simulink library "atlas_impctrl_library"  (Simulink 8.5)
settings: Solver=ode45  StartTime=0.0  StopTime=10.0  RelTol=1e-3
values from neighbouring files (symbols this model uses):
  B = d - 0.1*ones(NJL,1)    [atlas_joint_impctrl_sqrt_damping_test_settings_default.m]
  D = 0.7*eye(NJL)    [atlas_joint_impctrl_sqrt_damping_test_settings_default.m]
  K_d = 150*eye(NJL)    [atlas_joint_impctrl_sqrt_damping_test_settings_default.m]
  K_ext_c = 0    [atlas_joint_impctrl_sqrt_damping_test_settings_default.m]
  K_ext_o = 1    [atlas_joint_impctrl_sqrt_damping_test_settings_default.m]
  K_fri_o = 1    [atlas_joint_impctrl_sqrt_damping_test_settings_default.m]
  K_O = 5*eye(NJL)    [atlas_joint_impctrl_sqrt_damping_test_settings_default.m]
  K_obs_c = 0    [atlas_joint_impctrl_sqrt_damping_test_settings_default.m]
  K_qD_d = 1    [atlas_joint_impctrl_sqrt_damping_test_settings_default.m]
  K_qDD_d = 1    [atlas_joint_impctrl_sqrt_damping_test_settings_default.m]
  K_tau_a = 1    [atlas_joint_impctrl_sqrt_damping_test_settings_default.m]
  K_tau_c = 1    [atlas_joint_impctrl_sqrt_damping_test_settings_default.m]
  K_tau_D = 1    [atlas_joint_impctrl_sqrt_damping_test_settings_default.m]
  K_tau_e = 0    [atlas_joint_impctrl_sqrt_damping_test_settings_default.m]
  K_tau_f = 0    [atlas_joint_impctrl_sqrt_damping_test_settings_default.m]
  K_tau_g = 1    [atlas_joint_impctrl_sqrt_damping_test_settings_default.m]
  K_tau_K = 1    [atlas_joint_impctrl_sqrt_damping_test_settings_default.m]
  K_tau_o = 0    [atlas_joint_impctrl_sqrt_damping_test_settings_default.m]
  qD_th = 0.05*ones(NJL,1)    [atlas_joint_impctrl_sqrt_damping_test_settings_default.m]
  T = 0.001    [atlas_joint_impctrl_sqrt_damping_test_settings_default.m]
  T1 = 0    [atlas_joint_impctrl_sqrt_damping_test_settings_default.m]
  tau_c = muC - 4*ones(NJL,1)    [atlas_joint_impctrl_sqrt_damping_test_settings_default.m]
  tau_th = 0.02*ones(NJL,1)    [atlas_joint_impctrl_sqrt_damping_test_settings_default.m]
undefined symbols (not defined in the file or in its folder): K_tau_F, mr, offsets
undefined symbols (not defined in the file): atlas_arm_lr, atlas_leg_lr, delta_s, MPV, MPV_arm_damp, MPV_arm_model, MPV_leg_damp, MPV_leg_model, qD_s, tau_s
libraries: atlas_dynamic_library x23, atlas_impctrl_library x18, dspmtrx3 x3
(part 1 of 2)
settings Model: Creator=knoechelmann  LastModifiedBy=schappler  CovSFcnEnable=off

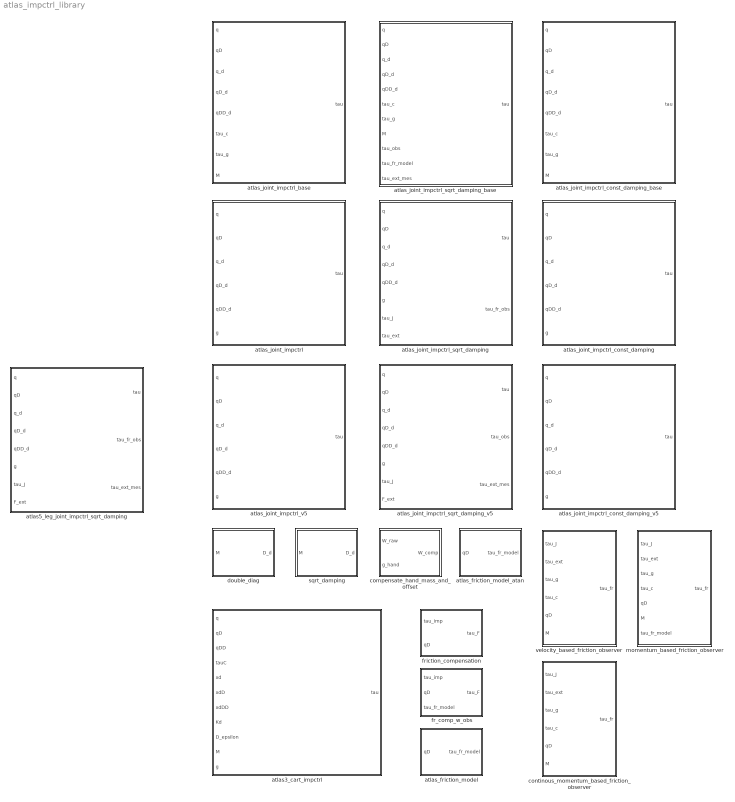
== system atlas_impctrl_library ==
  atlas3_cart_impctrl : Subsystem  TreatAsAtomicUnit=on
  atlas5_leg_joint_impctrl_sqrt_damping : Subsystem  TreatAsAtomicUnit=on  SystemSampleTime=T  mask(Atlas Joint Impedance Controller){K_d=K_d, D=D, K_tau_g=K_tau_g, K_tau_c=K_tau_c, K_tau_K=K_tau_K, K_tau_D=K_tau_D, K_tau_a=K_tau_a, K_tau_f=K_tau_f, K_tau_e=K_tau_e, K_tau_o=K_tau_o, K_qD_d=K_qD_d, K_qDD_d=K_qDD_d, K_ext_c=K_ext_c, K_obs_c=K_obs_c, K_fri_o=K_fri_o, K_ext_o=K_ext_o, tau_obs_max=30*ones(6,1), MPV_leg_damp=MPV_leg_damp, MPV_leg_model=MPV_leg_model, tau_c=tau_c, B=B, qD_th=qD_th, tau_th=tau_th, K_O=K_O, T=T, atlas_leg_lr=atlas_leg_lr, T1=T1}
      mask prompts: K_d "K_d (desired stiffness)"; D "D (diagonal matrix with desired damping coefficients)"; K_tau_g "K_tau_g (gain of gravity compensation)"; K_tau_c "K_tau_c (gain of corriolis- and inertia compensation)"; K_tau_K "K_tau_K (gain of stiffness component)"; K_tau_D "K_tau_D (gain of damping component)"; K_tau_a "K_tau_a (gain of acceleration component)"; K_tau_f "K_tau_f (gain of friction compensation)"; K_tau_e "K_tau_e (gain of external torque)"; K_tau_o "K_tau_o (gain of compensation of disturbance observer torques)"; K_qD_d "K_qD_d (gain of desired velocity)"; K_qDD_d "K_qDD_d (gain of desired acceleration)"; K_ext_c "K_ext_c (input gain to deside, wether to trigger friction compensation via the measured external torque)"; K_obs_c "K_obs_c (input gain to deside, wether to trigger friction compensation via the observed torque)"; K_fri_o "K_fri_o (input gain of friction model torques for observer)"; K_ext_o "K_ext_o (input gain of external torque for observer)"; tau_obs_max "tau_obs_max (limit for observed disturbance torque)"; MPV_leg_damp "MPV_damp (base parameter vector for damping calculation)"; MPV_leg_model "MPV_model (base parameter vector for dynamic model calculation)"; tau_c "tau_c (vector with coulomb friction momentums for all joints)"; B "B (vector with viscous friction coefficients of all joints)"; qD_th "qD_th (vector with theshold velocities for stiction)"; tau_th "tau_th (vector with kick-in momentums for stiction compensation)"; K_O "K_O (friction observer gain)"; T "T (sample time (important for friction observer))"; atlas_leg_lr "atlas_leg_lr (left/right flag)"; T1 "T1 (low pass filter time constant for inertia matrix)"
      mask help:
      | Hardware dependent full impedance controller block with matrix
      | squareroot damping design for the atlas robot. For a better
      | testing, all partial momentums can be individually scaled.
      | Coulomb-, viscous friction and Stribeck stiction is taken into
      | account for friction compensation.
  atlas_friction_model : Subsystem  TreatAsAtomicUnit=on  mask{tau_c=tau_c, B=B}
      mask prompts: tau_c "tau_c (vector with coulomb friction momentums for all joints)"; B "B (vector with viscous friction coefficients of all joints)"
  atlas_friction_model_atan : Subsystem  TreatAsAtomicUnit=on  mask{tau_c=tau_c, B=B}
      mask prompts: tau_c "tau_c (vector with coulomb friction momentums for all joints)"; B "B (vector with viscous friction coefficients of all joints)"
  atlas_joint_impctrl : Subsystem  TreatAsAtomicUnit=on  mask(Atlas Joint Impedance Controller){K_d=K_d, D=D, tau_c=tau_c, B=B, tau_s=tau_s, qD_s=qD_s, delta_s=delta_s, qD_th=qD_th, tau_th=tau_th, K_tau_g=K_tau_g, K_tau_c=K_tau_c, K_tau_F=K_tau_F, K_tau_K=K_tau_K, K_tau_D=K_tau_D, K_tau_a=K_tau_a, MPV=MPV}
      mask prompts: K_d "K_d (desired stiffness)"; D "D (diagonal matrix with desired damping coefficients)"; tau_c "tau_c (vector with coulomb friction momentums for all joints)"; B "B (vector with viscous friction coefficients of all joints)"; tau_s "tau_s (vector with sticition momentums of all joints)"; qD_s "qD_s (vector with Stribeck velocities of all joints)"; delta_s "delta_s (vector with stiction exponents for all joints)"; qD_th "qD_th (vector with theshold velocities for stiction)"; tau_th "tau_th (vector with kick-in momentums for stiction compensation)"; K_tau_g "K_tau_g (gain of gravity compensation)"; K_tau_c "K_tau_c (gain of corriolis- and inertia compensation)"; K_tau_F "K_tau_F (gain of friction compensation)"; K_tau_K "K_tau_K (gain of stiffness component)"; K_tau_D "K_tau_D (gain of damping component)"; K_tau_a "K_tau_a (gain of acceleration component)"; MPV "MPV (vector of minimal parameters)"
      mask help:
      | Hardware dependent full impedance controller block with matrix
      | double diagonalization damping design for the atlas robot. For
      | a better testing, all partial momentums can be individually
      | scaled. Coulomb-, viscous friction and Stribeck stiction is taken
      | into account for friction compensation.
  atlas_joint_impctrl_base : Subsystem  TreatAsAtomicUnit=on  mask(Joint Impedance Controller Base){K_d=K_d, D=D, tau_c=tau_c, B=B, tau_s=tau_s, qD_s=qD_s, delta_s=delta_s, qD_th=qD_th, tau_th=tau_th, K_tau_g=K_tau_g, K_tau_c=K_tau_c, K_tau_F=K_tau_F, K_tau_K=K_tau_K, K_tau_D=K_tau_D, K_tau_a=K_tau_a}
      mask prompts: K_d "K_d (desired stiffness)"; D "D (diagonal matrix with desired damping coefficients)"; tau_c "tau_c (vector with coulomb friction momentums for all joints)"; B "B (vector with viscous friction coefficients of all joints)"; tau_s "tau_s (vector with sticition momentums of all joints)"; qD_s "qD_s (vector with Stribeck velocities of all joints)"; delta_s "delta_s (vector with stiction exponents for all joints)"; qD_th "qD_th (vector with theshold velocities for stiction)"; tau_th "tau_th (vector with kick-in momentums for stiction compensation)"; K_tau_g "K_tau_g (gain of gravity compensation)"; K_tau_c "K_tau_c (gain of corriolis- and inertia compensation)"; K_tau_F "K_tau_F (gain of friction compensation)"; K_tau_K "K_tau_K (gain of stiffness component)"; K_tau_D "K_tau_D (gain of damping component)"; K_tau_a "K_tau_a (gain of acceleration component)"
      mask help:
      | Hardware independent impedance controller base block with mdouble
      | diagonalization damping design. For a better testing, all partial
      | momentums can be individually scaled. Coulomb-, viscous friction
      | and Stribeck stiction is taken into account for friction compen-
      | sation.
  atlas_joint_impctrl_const_damping : Subsystem  TreatAsAtomicUnit=on  mask(Atlas Joint Impedance Controller){K_d=K_d, D=D, tau_c=tau_c, B=B, tau_s=tau_s, qD_s=qD_s, delta_s=delta_s, qD_th=qD_th, tau_th=tau_th, K_tau_g=K_tau_g, K_tau_c=K_tau_c, K_tau_F=K_tau_F, K_tau_K=K_tau_K, K_tau_D=K_tau_D, K_tau_a=K_tau_a, MPV=MPV}
      mask prompts: K_d "K_d (desired stiffness)"; D "D (diagonal matrix with desired damping coefficients)"; tau_c "tau_c (vector with coulomb friction momentums for all joints)"; B "B (vector with viscous friction coefficients of all joints)"; tau_s "tau_s (vector with sticition momentums of all joints)"; qD_s "qD_s (vector with Stribeck velocities of all joints)"; delta_s "delta_s (vector with stiction exponents for all joints)"; qD_th "qD_th (vector with theshold velocities for stiction)"; tau_th "tau_th (vector with kick-in momentums for stiction compensation)"; K_tau_g "K_tau_g (gain of gravity compensation)"; K_tau_c "K_tau_c (gain of corriolis- and inertia compensation)"; K_tau_F "K_tau_F (gain of friction compensation)"; K_tau_K "K_tau_K (gain of stiffness component)"; K_tau_D "K_tau_D (gain of damping component)"; K_tau_a "K_tau_a (gain of acceleration component)"; MPV "MPV (vector of minimal parameters)"
      mask help:
      | Hardware dependent full impedance controller block with
      | constant damping design for the atlas robot. For a better
      | testing, all partial momentums can be individually scaled.
      | Coulomb-, viscous friction and Stribeck stiction is taken into
      | account for friction compensation.
  atlas_joint_impctrl_const_damping_base : Subsystem  TreatAsAtomicUnit=on  mask(Joint Impedance Controller Base){K_d=K_d, D=D, tau_c=tau_c, B=B, tau_s=tau_s, qD_s=qD_s, delta_s=delta_s, qD_th=qD_th, tau_th=tau_th, K_tau_g=K_tau_g, K_tau_c=K_tau_c, K_tau_F=K_tau_F, K_tau_K=K_tau_K, K_tau_D=K_tau_D, K_tau_a=K_tau_a}
      mask prompts: K_d "K_d (desired stiffness)"; D "D (diagonal matrix with desired damping coefficients)"; tau_c "tau_c (vector with coulomb friction momentums for all joints)"; B "B (vector with viscous friction coefficients of all joints)"; tau_s "tau_s (vector with sticition momentums of all joints)"; qD_s "qD_s (vector with Stribeck velocities of all joints)"; delta_s "delta_s (vector with stiction exponents for all joints)"; qD_th "qD_th (vector with theshold velocities for stiction)"; tau_th "tau_th (vector with kick-in momentums for stiction compensation)"; K_tau_g "K_tau_g (gain of gravity compensation)"; K_tau_c "K_tau_c (gain of corriolis- and inertia compensation)"; K_tau_F "K_tau_F (gain of friction compensation)"; K_tau_K "K_tau_K (gain of stiffness component)"; K_tau_D "K_tau_D (gain of damping component)"; K_tau_a "K_tau_a (gain of acceleration component)"
      mask help:
      | Hardware independent impedance controller base block with constant
      | damping design. For a better testing, all partial momentums can be
      | individually scaled. Coulomb-, viscous friction and Stribeck stiction
      | is taken into account for friction compensation.
  atlas_joint_impctrl_const_damping_v5 : Subsystem  TreatAsAtomicUnit=on  mask(Atlas Joint Impedance Controller){K_d=K_d, D=D, tau_c=tau_c, B=B, tau_s=tau_s, qD_s=qD_s, delta_s=delta_s, qD_th=qD_th, tau_th=tau_th, K_tau_g=K_tau_g, K_tau_c=K_tau_c, K_tau_F=K_tau_F, K_tau_K=K_tau_K, K_tau_D=K_tau_D, K_tau_a=K_tau_a, MPV=MPV}
      mask prompts: K_d "K_d (desired stiffness)"; D "D (diagonal matrix with desired damping coefficients)"; tau_c "tau_c (vector with coulomb friction momentums for all joints)"; B "B (vector with viscous friction coefficients of all joints)"; tau_s "tau_s (vector with sticition momentums of all joints)"; qD_s "qD_s (vector with Stribeck velocities of all joints)"; delta_s "delta_s (vector with stiction exponents for all joints)"; qD_th "qD_th (vector with theshold velocities for stiction)"; tau_th "tau_th (vector with kick-in momentums for stiction compensation)"; K_tau_g "K_tau_g (gain of gravity compensation)"; K_tau_c "K_tau_c (gain of corriolis- and inertia compensation)"; K_tau_F "K_tau_F (gain of friction compensation)"; K_tau_K "K_tau_K (gain of stiffness component)"; K_tau_D "K_tau_D (gain of damping component)"; K_tau_a "K_tau_a (gain of acceleration component)"; MPV "MPV (vector of minimal parameters)"
      mask help:
      | Hardware dependent full impedance controller block with
      | constant damping design for the atlas robot. For a better
      | testing, all partial momentums can be individually scaled.
      | Coulomb-, viscous friction and Stribeck stiction is taken into
      | account for friction compensation.
  atlas_joint_impctrl_sqrt_damping : Subsystem  TreatAsAtomicUnit=on  mask(Atlas Joint Impedance Controller){K_d=K_d, D=D, K_tau_g=K_tau_g, K_tau_c=K_tau_c, K_tau_K=K_tau_K, K_tau_D=K_tau_D, K_tau_a=K_tau_a, K_qD_d=K_qD_d, K_qDD_d=K_qDD_d, MPV=MPV, K_O=K_O, T=T}
      mask prompts: K_d "K_d (desired stiffness)"; D "D (diagonal matrix with desired damping coefficients)"; K_tau_g "K_tau_g (gain of gravity compensation)"; K_tau_c "K_tau_c (gain of corriolis- and inertia compensation)"; K_tau_K "K_tau_K (gain of stiffness component)"; K_tau_D "K_tau_D (gain of damping component)"; K_tau_a "K_tau_a (gain of acceleration component)"; K_qD_d "K_qD_d (gain of desired velocity)"; K_qDD_d "K_qDD_d (gain of desired acceleration)"; MPV "MPV (vector of minimal parameters)"; K_O "K_O (friction observer gain)"; T "T (sample time (important for friction observer))"
      mask help:
      | Hardware dependent full impedance controller block with matrix
      | squareroot damping design for the atlas robot. For a better
      | testing, all partial momentums can be individually scaled.
      | Coulomb-, viscous friction and Stribeck stiction is taken into
      | account for friction compensation.
  atlas_joint_impctrl_sqrt_damping_base : Subsystem  TreatAsAtomicUnit=on  mask(Joint Impedance Controller Base){K_d=K_d, D=D, K_tau_g=K_tau_g, K_tau_c=K_tau_c, K_tau_K=K_tau_K, K_tau_D=K_tau_D, K_tau_a=K_tau_a, K_tau_f=K_tau_f, K_tau_e=K_tau_e, K_tau_o=K_tau_o, K_qD_d=K_qD_d, K_qDD_d=K_qDD_d, K_ext_c=K_ext_c, K_obs_c=K_obs_c, tau_c=tau_c, B=B, qD_th=qD_th, tau_th=tau_th}
      mask prompts: K_d "K_d (desired stiffness)"; D "D (diagonal matrix with desired damping coefficients)"; K_tau_g "K_tau_g (gain of gravity compensation)"; K_tau_c "K_tau_c (gain of corriolis- and inertia compensation)"; K_tau_K "K_tau_K (gain of stiffness component)"; K_tau_D "K_tau_D (gain of damping component)"; K_tau_a "K_tau_a (gain of acceleration component)"; K_tau_f "K_tau_f (gain of model based friction compensation)"; K_tau_e "K_tau_e (gain of compensation of external torque measurd via hand sensor)"; K_tau_o "K_tau_o (gain of compensation of disturbance observer torques)"; K_qD_d "K_qD_d (gain of desired velocity)"; K_qDD_d "K_qDD_d (gain of desired acceleration)"; K_ext_c "K_ext_c (input gain to deside, wether to trigger friction compensation via the measured external torque)"; K_obs_c "K_obs_c (input gain to deside, wether to trigger friction compensation via the observed torque)"; tau_c "tau_c (vector with coulomb friction momentums for all joints)"; B "B (vector with viscous friction coefficients of all joints)"; qD_th "qD_th (vector with theshold velocities for stiction)"; tau_th "tau_th (vector with kick-in momentums for stiction compensation)"
      mask help:
      | Hardware independent impedance controller base block with matrix
      | squareroot damping design. For a better testing, all partial mo-
      | mentums can be individually scaled. Coulomb-, viscous friction
      | and Stribeck stiction is taken into account for friction compen-
      | sation.
  atlas_joint_impctrl_sqrt_damping_v5 : Subsystem  TreatAsAtomicUnit=on  SystemSampleTime=T  mask(Atlas Joint Impedance Controller){K_d=K_d, D=D, K_tau_g=K_tau_g, K_tau_c=K_tau_c, K_tau_K=K_tau_K, K_tau_D=K_tau_D, K_tau_a=K_tau_a, K_tau_f=K_tau_f, K_tau_e=K_tau_e, K_tau_o=K_tau_o, K_qD_d=K_qD_d, K_qDD_d=K_qDD_d, K_ext_c=K_ext_c, K_obs_c=K_obs_c, K_fri_o=K_fri_o, K_ext_o=K_ext_o, tau_obs_max=30*ones(7,1), MPV_arm_damp=MPV_arm_damp, MPV_arm_model=MPV_arm_model, tau_c=tau_c, B=B, qD_th=qD_th, tau_th=tau_th, K_O=K_O, T=T, atlas_arm_lr=atlas_arm_lr, T1=T1}
      mask prompts: K_d "K_d (desired stiffness)"; D "D (diagonal matrix with desired damping coefficients)"; K_tau_g "K_tau_g (gain of gravity compensation)"; K_tau_c "K_tau_c (gain of corriolis- and inertia compensation)"; K_tau_K "K_tau_K (gain of stiffness component)"; K_tau_D "K_tau_D (gain of damping component)"; K_tau_a "K_tau_a (gain of acceleration component)"; K_tau_f "K_tau_f (gain of model based friction compensation)"; K_tau_e "K_tau_e (gain of compensation of external torque measurd via hand sensor)"; K_tau_o "K_tau_o (gain of compensation of disturbance observer torques)"; K_qD_d "K_qD_d (gain of desired velocity)"; K_qDD_d "K_qDD_d (gain of desired acceleration)"; K_ext_c "K_ext_c (input gain to deside, wether to trigger friction compensation via the measured external torque)"; K_obs_c "K_obs_c (input gain to deside, wether to trigger friction compensation via the observed torque)"; K_fri_o "K_fri_o (input gain of friction model torques for observer)"; K_ext_o "K_ext_o (input gain of external torque for observer)"; tau_obs_max "tau_obs_max (limit for observed disturbance torque)"; MPV_arm_damp "MPV_damp (base parameter vector for damping calculation)"; MPV_arm_model "MPV_model (base parameter vector for dynamic model calculation)"; tau_c "tau_c (vector with coulomb friction momentums for all joints)"; B "B (vector with viscous friction coefficients of all joints)"; qD_th "qD_th (vector with theshold velocities for stiction)"; tau_th "tau_th (vector with kick-in momentums for stiction compensation)"; K_O "K_O (friction observer gain)"; T "T (sample time (important for friction observer))"; atlas_arm_lr "atlas_arm_lr (flag for left or right side)"; T1 "T1 (low pass filter time constant for inertia matrix)"
      mask help:
      | Hardware dependent full impedance controller block with matrix
      | squareroot damping design for the atlas robot. For a better
      | testing, all partial momentums can be individually scaled.
      | Coulomb-, viscous friction and Stribeck stiction is taken into
      | account for friction compensation.
  atlas_joint_impctrl_v5 : Subsystem  TreatAsAtomicUnit=on  mask(Atlas Joint Impedance Controller){K_d=K_d, D=D, tau_c=tau_c, B=B, tau_s=tau_s, qD_s=qD_s, delta_s=delta_s, qD_th=qD_th, tau_th=tau_th, K_tau_g=K_tau_g, K_tau_c=K_tau_c, K_tau_F=K_tau_F, K_tau_K=K_tau_K, K_tau_D=K_tau_D, K_tau_a=K_tau_a, MPV=MPV}
      mask prompts: K_d "K_d (desired stiffness)"; D "D (diagonal matrix with desired damping coefficients)"; tau_c "tau_c (vector with coulomb friction momentums for all joints)"; B "B (vector with viscous friction coefficients of all joints)"; tau_s "tau_s (vector with sticition momentums of all joints)"; qD_s "qD_s (vector with Stribeck velocities of all joints)"; delta_s "delta_s (vector with stiction exponents for all joints)"; qD_th "qD_th (vector with theshold velocities for stiction)"; tau_th "tau_th (vector with kick-in momentums for stiction compensation)"; K_tau_g "K_tau_g (gain of gravity compensation)"; K_tau_c "K_tau_c (gain of corriolis- and inertia compensation)"; K_tau_F "K_tau_F (gain of friction compensation)"; K_tau_K "K_tau_K (gain of stiffness component)"; K_tau_D "K_tau_D (gain of damping component)"; K_tau_a "K_tau_a (gain of acceleration component)"; MPV "MPV (vector of minimal parameters)"
      mask help:
      | Hardware dependent full impedance controller block with matrix
      | double diagonalization damping design for the atlas robot. For
      | a better testing, all partial momentums can be individually
      | scaled. Coulomb-, viscous friction and Stribeck stiction is taken
      | into account for friction compensation.
  compensate_hand_mass_and_offset : Subsystem  TreatAsAtomicUnit=on  mask{mr=mr, Parameter2offsets=offsets}
      mask prompts: mr "mr (mass (1) and com  (2-4) of the hand in hand frame)"; Parameter2offsets "offsets (sensor offsets of F/T-sensor)"
  continous_momentum_based_friction_observer : Subsystem  TreatAsAtomicUnit=on  mask{K_O=K_O}
      mask prompts: K_O "K_O (Observer gain)"
  double_diag : Subsystem  TreatAsAtomicUnit=on  mask{K_d=K_d, D=D}
  fr_comp_w_obs : Subsystem  TreatAsAtomicUnit=on  mask{tau_c=tau_c, B=B, qD_th=qD_th, tau_th=tau_th}
      mask prompts: tau_c "tau_c (vector with coulomb friction momentums for all joints)"; B "B (vector with viscous friction coefficients of all joints)"; qD_th "qD_th (vector with theshold velocities for stiction)"; tau_th "tau_th (vector with kick-in momentums for stiction compensation)"
  friction_compensation : Subsystem  TreatAsAtomicUnit=on  mask{tau_c=tau_c, B=B, qD_th=qD_th, tau_th=tau_th}
      mask prompts: tau_c "tau_c (vector with coulomb friction momentums for all joints)"; B "B (vector with viscous friction coefficients of all joints)"; qD_th "qD_th (vector with theshold velocities for stiction)"; tau_th "tau_th (vector with kick-in momentums for stiction compensation)"
  momentum_based_friction_observer : Subsystem  TreatAsAtomicUnit=on  SystemSampleTime=T  mask{K_O=K_O, T=T, T1=T1, tau_out_max=30*ones(6,1)}
      mask prompts: K_O "K_O (Observer gain)"; T "T (sampletime)"; T1 "T1 (low pass differentiator time constant)"; tau_out_max "tau_out_max (safety limit for output, output will be limited to lie in between -tau_out_max and tau_out_max)"
  sqrt_damping : Subsystem  TreatAsAtomicUnit=on  mask{K_d=K_d, D=D}
  velocity_based_friction_observer : Subsystem  TreatAsAtomicUnit=on  mask{K_O=K_O, T=T}
      mask prompts: K_O "K_O (Observer gain)"; T "T (sampletime)"

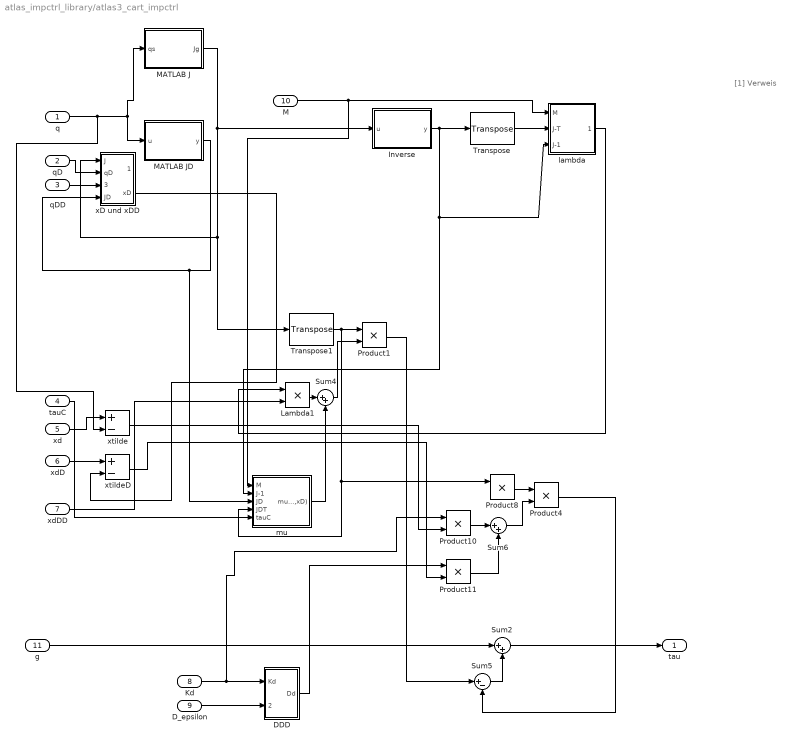
== system atlas_impctrl_library/atlas3_cart_impctrl ==
  note: [1] Verweis
  q : Inport
  qD : Inport  Port=2
  qDD : Inport  Port=3
  tauC : Inport  Port=4
  xd : Inport  Port=5
  xdD : Inport  Port=6
  xdDD : Inport  Port=7
  Kd : Inport  Port=8
  D_epsilon : Inport  Port=9
  M : Inport  Port=10
  g : Inport  Port=11
  DDD : Subsystem
  Inverse : MATLAB Function  TreatAsAtomicUnit=on
  Lambda1 : Product
  MATLAB J : MATLAB Function  TreatAsAtomicUnit=on
  MATLAB JD : MATLAB Function  TreatAsAtomicUnit=on
  Product{1,4,8,10..11} (5 alike) : Product
  Sum2 : Sum  Inputs=|++
  Sum4 : Sum  Inputs=|++
  Sum5 : Sum  Inputs=|+-
  Sum6 : Sum  Inputs=|++
  Transpose : dspmtrx3/Transpose  Hermitian=off  overflowFlag=off
  Transpose1 : dspmtrx3/Transpose  Hermitian=off  overflowFlag=off
  lambda : Subsystem
  mu : Subsystem
  xD und xDD : Subsystem
  xtilde : Sum  Inputs=+-
  xtildeD : Sum  Inputs=+-
  tau : Outport
  wires:
  DDD/1(Dd) -> Product11/1
  Product10/1 -> Sum6/1
  Product8/1 -> Product4/1
  xdD/1 -> xtildeD/1
  Transpose1/1 -> Product8/1, mu/4(JDT), Product1/1
  Product4/1 -> Sum5/2
  Product11/1 -> Sum6/2
  Sum2/1 -> tau/1
  Inverse/1(y) -> mu/2(J-1), lambda/3(J-1), Transpose/1
  g/1 -> Sum2/1
  Sum6/1 -> Product4/2
  M/1 -> mu/1(M), lambda/1(M)
  MATLAB J/1(Jg) -> xD und xDD/1(J), Transpose1/1, Inverse/1(u)
  xd/1 -> xtilde/1
  xtilde/1 -> Product10/2
  MATLAB JD/1(y) -> mu/3(JD), xD und xDD/4(JD)
  Sum4/1 -> Product1/2
  Sum5/1 -> Sum2/2
  Lambda1/1 -> Sum4/1
  xdDD/1 -> Lambda1/2
  q/1 -> MATLAB J/1(qs), MATLAB JD/1(u), xtilde/2
  xtildeD/1 -> Product11/2
  Product1/1 -> Sum5/1
  lambda/1(Lambda) -> Lambda1/1
  Transpose/1 -> lambda/2(J-T)
  tauC/1 -> mu/5(tauC)
  mu/1(mu(x,xD)) -> Sum4/2
  qD/1 -> xD und xDD/2(qD)
  qDD/1 -> xD und xDD/3(qDD)
  xD und xDD/2(xD) -> xtildeD/2
  Kd/1 -> Product10/1, DDD/1(Kd)
  D_epsilon/1 -> DDD/2(D_epsilon)

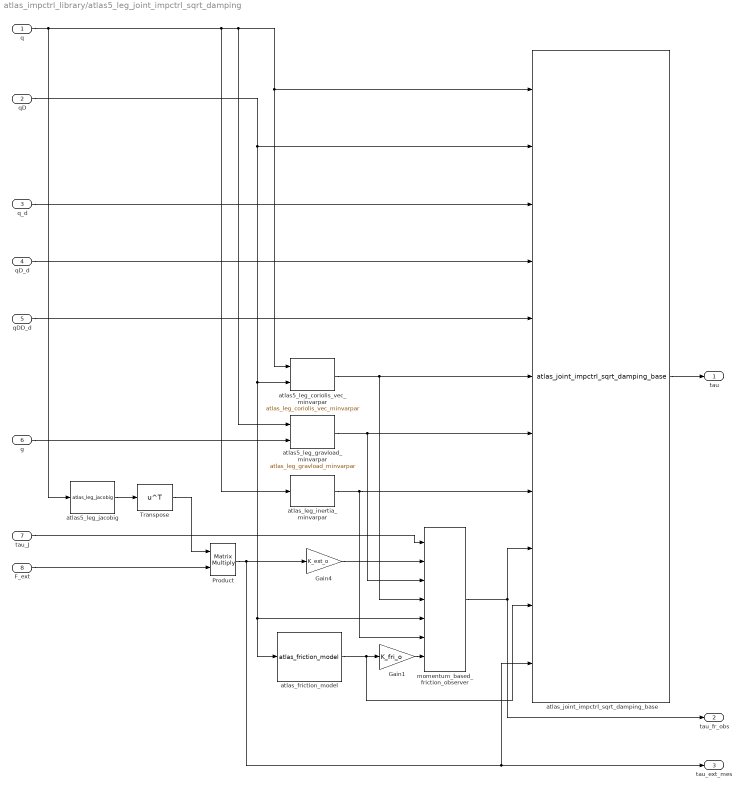
== system atlas_impctrl_library/atlas5_leg_joint_impctrl_sqrt_damping ==
  q : Inport  OutDataTypeStr=double  PortDimensions=6
  qD : Inport  Port=2  OutDataTypeStr=double  PortDimensions=6
  q_d : Inport  Port=3  OutDataTypeStr=double  PortDimensions=6
  qD_d : Inport  Port=4  OutDataTypeStr=double  PortDimensions=6
  qDD_d : Inport  Port=5  OutDataTypeStr=double  PortDimensions=6
  g : Inport  Port=6  OutDataTypeStr=double  PortDimensions=[3 1]
  tau_J : Inport  Port=7  OutDataTypeStr=double  PortDimensions=6
  F_ext : Inport  Port=8  OutDataTypeStr=double  PortDimensions=6
  Gain1 : Gain  Gain=K_fri_o
  Gain4 : Gain  Gain=K_ext_o
  Product : Product  Multiplication=Matrix(*)
  Transpose : Math  Operator=transpose  SaturateOnIntegerOverflow=on
  atlas5_leg_coriolis_vec_minvarpar : atlas_dynamic_library/atlas_leg_coriolis_vec_minvarpar  atlas_arm_lr=atlas_leg_lr  atlas_version=uint8(5)  MPV=MPV_leg_model
  atlas5_leg_gravload_minvarpar : atlas_dynamic_library/atlas_leg_gravload_minvarpar  atlas_arm_lr=atlas_leg_lr  atlas_version=uint8(5)  MPV=MPV_leg_model
  atlas5_leg_jacobig : atlas_dynamic_library/atlas_leg_jacobig  atlas_version=uint8(5)  atlas_leg_lr=atlas_leg_lr
  atlas_friction_model : atlas_impctrl_library/atlas_friction_model  tau_c=tau_c  B=B
  atlas_joint_impctrl_sqrt_damping_base : atlas_impctrl_library/atlas_joint_impctrl_sqrt_damping_base  K_d=K_d  D=D  K_tau_g=K_tau_g  K_tau_c=K_tau_c  K_tau_K=K_tau_K  K_tau_D=K_tau_D  K_tau_a=K_tau_a  K_tau_f=K_tau_f  K_tau_e=K_tau_e  K_tau_o=K_tau_o  K_qD_d=K_qD_d  K_qDD_d=K_qDD_d  K_ext_c=K_ext_c  K_obs_c=K_obs_c  tau_c=tau_c  B=B  qD_th=qD_th  tau_th=tau_th
  atlas_leg_inertia_minvarpar : atlas_dynamic_library/atlas_leg_inertia_minvarpar  atlas_arm_lr=atlas_leg_lr  atlas_version=uint8(5)  MPV=MPV_leg_damp
  momentum_based_friction_observer : atlas_impctrl_library/momentum_based_friction_observer  K_O=K_O  T=T  T1=T1  tau_out_max=tau_obs_max
  tau : Outport  OutDataTypeStr=double  PortDimensions=6
  tau_fr_obs : Outport  Port=2  OutDataTypeStr=double  PortDimensions=6
  tau_ext_mes : Outport  Port=3  OutDataTypeStr=double  PortDimensions=6
  wires:
  atlas_joint_impctrl_sqrt_damping_base/1 -> tau/1
  atlas_leg_inertia_minvarpar/1 -> atlas_joint_impctrl_sqrt_damping_base/8, momentum_based_friction_observer/6
  q/1 -> atlas_joint_impctrl_sqrt_damping_base/1, atlas5_leg_coriolis_vec_minvarpar/1, atlas5_leg_gravload_minvarpar/1, atlas_leg_inertia_minvarpar/1, atlas5_leg_jacobig/1
  qD/1 -> atlas_joint_impctrl_sqrt_damping_base/2, atlas5_leg_coriolis_vec_minvarpar/2, momentum_based_friction_observer/5, atlas_friction_model/1
  q_d/1 -> atlas_joint_impctrl_sqrt_damping_base/3
  atlas5_leg_coriolis_vec_minvarpar/1 -> atlas_joint_impctrl_sqrt_damping_base/6, momentum_based_friction_observer/4
  qD_d/1 -> atlas_joint_impctrl_sqrt_damping_base/4
  atlas5_leg_gravload_minvarpar/1 -> atlas_joint_impctrl_sqrt_damping_base/7, momentum_based_friction_observer/3
  qDD_d/1 -> atlas_joint_impctrl_sqrt_damping_base/5
  g/1 -> atlas5_leg_gravload_minvarpar/2
  momentum_based_friction_observer/1 -> tau_fr_obs/1, atlas_joint_impctrl_sqrt_damping_base/9
  tau_J/1 -> momentum_based_friction_observer/1
  atlas5_leg_jacobig/1 -> Transpose/1
  Transpose/1 -> Product/1
  F_ext/1 -> Product/2
  Product/1 -> atlas_joint_impctrl_sqrt_damping_base/11, tau_ext_mes/1, Gain4/1
  Gain4/1 -> momentum_based_friction_observer/2
  atlas_friction_model/1 -> atlas_joint_impctrl_sqrt_damping_base/10, Gain1/1
  Gain1/1 -> momentum_based_friction_observer/7

== system atlas_impctrl_library/atlas_friction_model ==
  qD : Inport
  atlas_friction_model : MATLAB Function  TreatAsAtomicUnit=on
  tau_fr_model : Outport
  wires:
  qD/1 -> atlas_friction_model/1(qD)
  atlas_friction_model/1(tau_fr_model) -> tau_fr_model/1

== system atlas_impctrl_library/atlas_friction_model_atan ==
  qD : Inport
  atlas_friction_model_atan : MATLAB Function  TreatAsAtomicUnit=on
  tau_fr_model : Outport
  wires:
  qD/1 -> atlas_friction_model_atan/1(qD)
  atlas_friction_model_atan/1(tau_fr_model) -> tau_fr_model/1

== system atlas_impctrl_library/atlas_joint_impctrl ==
  q : Inport
  qD : Inport  Port=2
  q_d : Inport  Port=3
  qD_d : Inport  Port=4
  qDD_d : Inport  Port=5
  g : Inport  Port=6
  atlas_arm_coriolis_vec_minvarpar : atlas_dynamic_library/atlas_arm_coriolis_vec_minvarpar  atlas_arm_lr=atlas_arm_lr  atlas_version=atlas_version  MPV=MPV
  atlas_arm_gravload_minvarpar : atlas_dynamic_library/atlas_arm_gravload_minvarpar  atlas_arm_lr=atlas_arm_lr  atlas_version=atlas_version  MPV=MPV
  atlas_arm_inertia_minvarpar : atlas_dynamic_library/atlas_arm_inertia_minvarpar  atlas_arm_lr=atlas_arm_lr  atlas_version=atlas_version  MPV=MPV
  atlas_joint_impctrl_base : atlas_impctrl_library/atlas_joint_impctrl_base  K_d=K_d  D=D  tau_c=tau_c  B=B  tau_s=tau_s  qD_s=qD_s  delta_s=delta_s  qD_th=qD_th  tau_th=tau_th  K_tau_g=K_tau_g  K_tau_c=K_tau_c  K_tau_F=K_tau_F  K_tau_K=K_tau_K  K_tau_D=K_tau_D  K_tau_a=K_tau_a
  tau : Outport
  wires:
  atlas_joint_impctrl_base/1 -> tau/1
  atlas_arm_inertia_minvarpar/1 -> atlas_joint_impctrl_base/8
  q/1 -> atlas_arm_inertia_minvarpar/1, atlas_arm_gravload_minvarpar/1, atlas_joint_impctrl_base/1, atlas_arm_coriolis_vec_minvarpar/1
  qD/1 -> atlas_joint_impctrl_base/2, atlas_arm_coriolis_vec_minvarpar/2
  q_d/1 -> atlas_joint_impctrl_base/3
  atlas_arm_coriolis_vec_minvarpar/1 -> atlas_joint_impctrl_base/6
  qD_d/1 -> atlas_joint_impctrl_base/4
  atlas_arm_gravload_minvarpar/1 -> atlas_joint_impctrl_base/7
  qDD_d/1 -> atlas_joint_impctrl_base/5
  g/1 -> atlas_arm_gravload_minvarpar/2

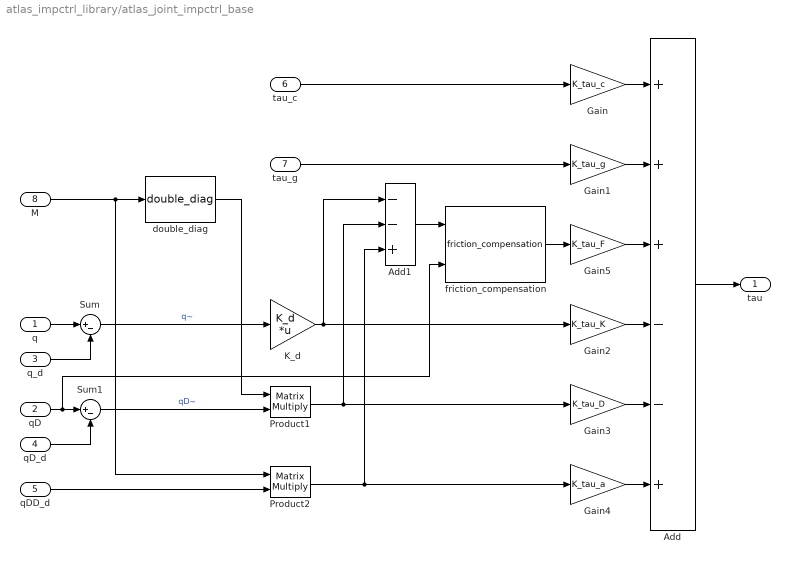
== system atlas_impctrl_library/atlas_joint_impctrl_base ==
  q : Inport
  qD : Inport  Port=2
  q_d : Inport  Port=3
  qD_d : Inport  Port=4
  qDD_d : Inport  Port=5
  tau_c : Inport  Port=6
  tau_g : Inport  Port=7
  M : Inport  Port=8
  Add : Sum  Inputs=+++--+
  Add1 : Sum  Inputs=--+
  Gain : Gain  Gain=K_tau_c
  Gain1 : Gain  Gain=K_tau_g
  Gain2 : Gain  Gain=K_tau_K
  Gain3 : Gain  Gain=K_tau_D
  Gain4 : Gain  Gain=K_tau_a
  Gain5 : Gain  Gain=K_tau_F
  K_d : Gain  Gain=K_d  Multiplication=Matrix(K*u)
  Product1 : Product  Multiplication=Matrix(*)
  Product2 : Product  Multiplication=Matrix(*)
  Sum : Sum  Inputs=|+-
  Sum1 : Sum  Inputs=|+-
  double_diag : atlas_impctrl_library/double_diag  K_d=K_d  D=D
  friction_compensation : atlas_impctrl_library/friction_compensation  tau_c=tau_c  B=B  qD_th=qD_th  tau_th=tau_th
  tau : Outport
  wires:
  M/1 -> double_diag/1, Product2/1
  q/1 -> Sum/1
  q_d/1 -> Sum/2
  qD/1 -> friction_compensation/2, Sum1/1
  qD_d/1 -> Sum1/2
  Sum1/1 -> Product1/2  "qD~"
  Sum/1 -> K_d/1  "q~"
  qDD_d/1 -> Product2/2
  double_diag/1 -> Product1/1
  Add/1 -> tau/1
  K_d/1 -> Add1/1, Gain2/1
  tau_g/1 -> Gain1/1
  tau_c/1 -> Gain/1
  Product1/1 -> Add1/2, Gain3/1
  Product2/1 -> Add1/3, Gain4/1
  Gain/1 -> Add/1
  Gain1/1 -> Add/2
  Gain2/1 -> Add/4
  Gain3/1 -> Add/5
  Gain4/1 -> Add/6
  Gain5/1 -> Add/3
  friction_compensation/1 -> Gain5/1
  Add1/1 -> friction_compensation/1

== system atlas_impctrl_library/atlas_joint_impctrl_const_damping ==
  q : Inport
  qD : Inport  Port=2
  q_d : Inport  Port=3
  qD_d : Inport  Port=4
  qDD_d : Inport  Port=5
  g : Inport  Port=6
  atlas_arm_coriolis_vec_minvarpar : atlas_dynamic_library/atlas_arm_coriolis_vec_minvarpar  atlas_arm_lr=atlas_arm_lr  atlas_version=atlas_version  MPV=MPV
  atlas_arm_gravload_minvarpar : atlas_dynamic_library/atlas_arm_gravload_minvarpar  atlas_arm_lr=atlas_arm_lr  atlas_version=atlas_version  MPV=MPV
  atlas_arm_inertia_minvarpar : atlas_dynamic_library/atlas_arm_inertia_minvarpar  atlas_arm_lr=atlas_arm_lr  atlas_version=atlas_version  MPV=MPV
  atlas_joint_impctrl_const_damping_base : atlas_impctrl_library/atlas_joint_impctrl_const_damping_base  K_d=K_d  D=D  tau_c=tau_c  B=B  tau_s=tau_s  qD_s=qD_s  delta_s=delta_s  qD_th=qD_th  tau_th=tau_th  K_tau_g=K_tau_g  K_tau_c=K_tau_c  K_tau_F=K_tau_F  K_tau_K=K_tau_K  K_tau_D=K_tau_D  K_tau_a=K_tau_a
  tau : Outport
  wires:
  atlas_joint_impctrl_const_damping_base/1 -> tau/1
  atlas_arm_inertia_minvarpar/1 -> atlas_joint_impctrl_const_damping_base/8
  q/1 -> atlas_arm_inertia_minvarpar/1, atlas_arm_gravload_minvarpar/1, atlas_joint_impctrl_const_damping_base/1, atlas_arm_coriolis_vec_minvarpar/1
  qD/1 -> atlas_joint_impctrl_const_damping_base/2, atlas_arm_coriolis_vec_minvarpar/2
  q_d/1 -> atlas_joint_impctrl_const_damping_base/3
  atlas_arm_coriolis_vec_minvarpar/1 -> atlas_joint_impctrl_const_damping_base/6
  qD_d/1 -> atlas_joint_impctrl_const_damping_base/4
  atlas_arm_gravload_minvarpar/1 -> atlas_joint_impctrl_const_damping_base/7
  qDD_d/1 -> atlas_joint_impctrl_const_damping_base/5
  g/1 -> atlas_arm_gravload_minvarpar/2

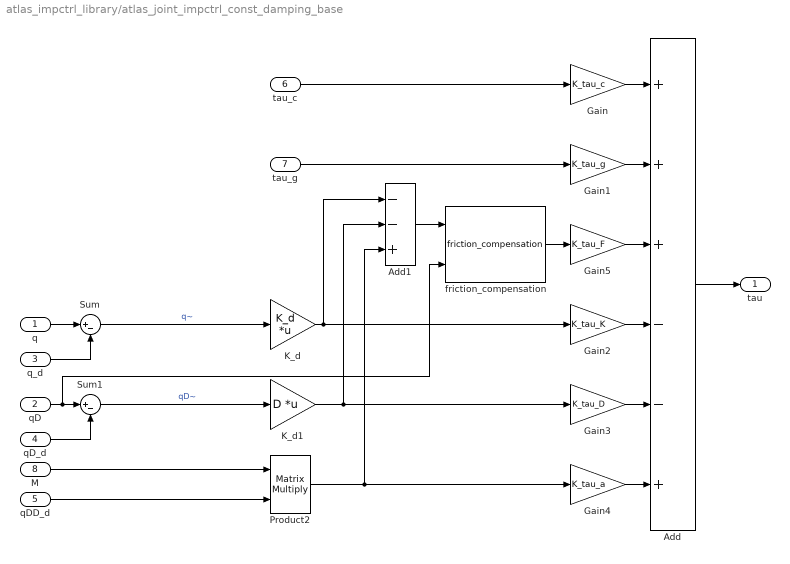
== system atlas_impctrl_library/atlas_joint_impctrl_const_damping_base ==
  q : Inport
  qD : Inport  Port=2
  q_d : Inport  Port=3
  qD_d : Inport  Port=4
  qDD_d : Inport  Port=5
  tau_c : Inport  Port=6
  tau_g : Inport  Port=7
  M : Inport  Port=8
  Add : Sum  Inputs=+++--+
  Add1 : Sum  Inputs=--+
  Gain : Gain  Gain=K_tau_c
  Gain1 : Gain  Gain=K_tau_g
  Gain2 : Gain  Gain=K_tau_K
  Gain3 : Gain  Gain=K_tau_D
  Gain4 : Gain  Gain=K_tau_a
  Gain5 : Gain  Gain=K_tau_F
  K_d : Gain  Gain=K_d  Multiplication=Matrix(K*u)
  K_d1 : Gain  Gain=D  Multiplication=Matrix(K*u)
  Product2 : Product  Multiplication=Matrix(*)
  Sum : Sum  Inputs=|+-
  Sum1 : Sum  Inputs=|+-
  friction_compensation : atlas_impctrl_library/friction_compensation  tau_c=tau_c  B=B  qD_th=qD_th  tau_th=tau_th
  tau : Outport
  wires:
  M/1 -> Product2/1
  q/1 -> Sum/1
  q_d/1 -> Sum/2
  qD/1 -> friction_compensation/2, Sum1/1
  qD_d/1 -> Sum1/2
  Sum1/1 -> K_d1/1  "qD~"
  Sum/1 -> K_d/1  "q~"
  qDD_d/1 -> Product2/2
  Add/1 -> tau/1
  K_d/1 -> Add1/1, Gain2/1
  tau_g/1 -> Gain1/1
  tau_c/1 -> Gain/1
  K_d1/1 -> Add1/2, Gain3/1
  Product2/1 -> Add1/3, Gain4/1
  Gain/1 -> Add/1
  Gain1/1 -> Add/2
  Gain2/1 -> Add/4
  Gain3/1 -> Add/5
  Gain4/1 -> Add/6
  Gain5/1 -> Add/3
  friction_compensation/1 -> Gain5/1
  Add1/1 -> friction_compensation/1

== system atlas_impctrl_library/atlas_joint_impctrl_const_damping_v5 ==
  q : Inport
  qD : Inport  Port=2
  q_d : Inport  Port=3
  qD_d : Inport  Port=4
  qDD_d : Inport  Port=5
  g : Inport  Port=6
  atlas_arm_coriolis_vec_minvarpar : atlas_dynamic_library/atlas_arm_coriolis_vec_minvarpar  atlas_arm_lr=atlas_arm_lr  atlas_version=atlas_version  MPV=MPV
  atlas_arm_gravload_minvarpar : atlas_dynamic_library/atlas_arm_gravload_minvarpar  atlas_arm_lr=atlas_arm_lr  atlas_version=atlas_version  MPV=MPV
  atlas_arm_inertia_minvarpar : atlas_dynamic_library/atlas_arm_inertia_minvarpar  atlas_arm_lr=atlas_arm_lr  atlas_version=atlas_version  MPV=MPV
  atlas_joint_impctrl_const_damping_base : atlas_impctrl_library/atlas_joint_impctrl_const_damping_base  K_d=K_d  D=D  tau_c=tau_c  B=B  tau_s=tau_s  qD_s=qD_s  delta_s=delta_s  qD_th=qD_th  tau_th=tau_th  K_tau_g=K_tau_g  K_tau_c=K_tau_c  K_tau_F=K_tau_F  K_tau_K=K_tau_K  K_tau_D=K_tau_D  K_tau_a=K_tau_a
  tau : Outport
  wires:
  atlas_joint_impctrl_const_damping_base/1 -> tau/1
  atlas_arm_inertia_minvarpar/1 -> atlas_joint_impctrl_const_damping_base/8
  q/1 -> atlas_arm_inertia_minvarpar/1, atlas_arm_gravload_minvarpar/1, atlas_joint_impctrl_const_damping_base/1, atlas_arm_coriolis_vec_minvarpar/1
  qD/1 -> atlas_joint_impctrl_const_damping_base/2, atlas_arm_coriolis_vec_minvarpar/2
  q_d/1 -> atlas_joint_impctrl_const_damping_base/3
  atlas_arm_coriolis_vec_minvarpar/1 -> atlas_joint_impctrl_const_damping_base/6
  qD_d/1 -> atlas_joint_impctrl_const_damping_base/4
  atlas_arm_gravload_minvarpar/1 -> atlas_joint_impctrl_const_damping_base/7
  qDD_d/1 -> atlas_joint_impctrl_const_damping_base/5
  g/1 -> atlas_arm_gravload_minvarpar/2

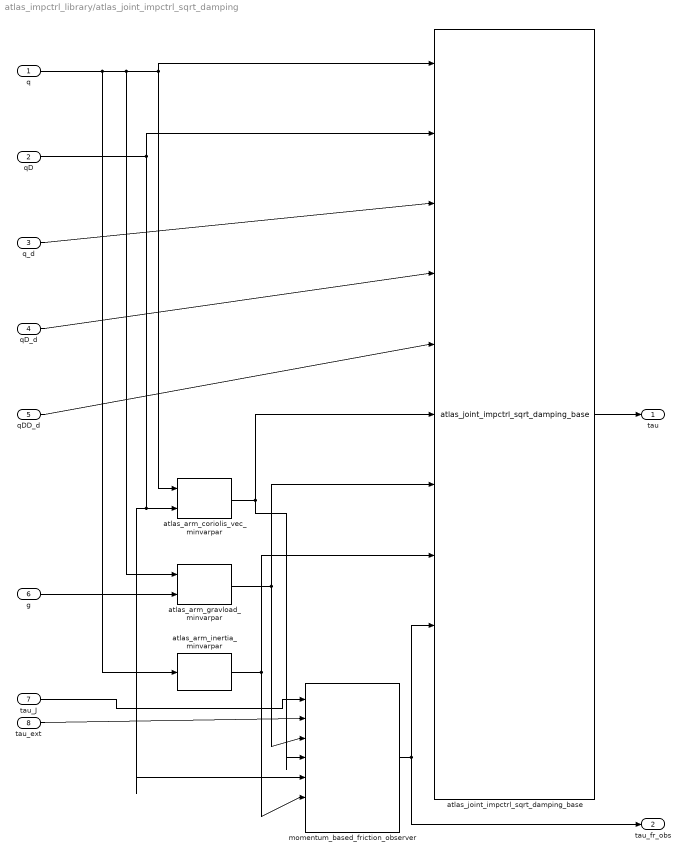
== system atlas_impctrl_library/atlas_joint_impctrl_sqrt_damping ==
  q : Inport
  qD : Inport  Port=2
  q_d : Inport  Port=3
  qD_d : Inport  Port=4
  qDD_d : Inport  Port=5
  g : Inport  Port=6
  tau_J : Inport  Port=7
  tau_ext : Inport  Port=8
  atlas_arm_coriolis_vec_minvarpar : atlas_dynamic_library/atlas_arm_coriolis_vec_minvarpar  atlas_arm_lr=atlas_arm_lr  atlas_version=atlas_version  MPV=MPV
  atlas_arm_gravload_minvarpar : atlas_dynamic_library/atlas_arm_gravload_minvarpar  atlas_arm_lr=atlas_arm_lr  atlas_version=atlas_version  MPV=MPV
  atlas_arm_inertia_minvarpar : atlas_dynamic_library/atlas_arm_inertia_minvarpar  atlas_arm_lr=atlas_arm_lr  atlas_version=atlas_version  MPV=MPV
  atlas_joint_impctrl_sqrt_damping_base : atlas_impctrl_library/atlas_joint_impctrl_sqrt_damping_base  K_d=K_d  D=D  K_tau_g=K_tau_g  K_tau_c=K_tau_c  K_tau_K=K_tau_K  K_tau_D=K_tau_D  K_tau_a=K_tau_a  K_tau_f=K_tau_F  K_tau_e=K_tau_e  K_tau_o=K_tau_o  K_qD_d=K_qD_d  K_qDD_d=K_qDD_d  K_ext_c=K_ext_c  K_obs_c=K_obs_c  tau_c=tau_c  B=B  qD_th=qD_th  tau_th=tau_th
  momentum_based_friction_observer : atlas_impctrl_library/momentum_based_friction_observer  K_O=K_O  T=T  T1=T1  tau_out_max=30*ones(7,1)
  tau : Outport
  tau_fr_obs : Outport  Port=2
  wires:
  atlas_joint_impctrl_sqrt_damping_base/1 -> tau/1
  atlas_arm_inertia_minvarpar/1 -> momentum_based_friction_observer/6, atlas_joint_impctrl_sqrt_damping_base/8
  q/1 -> atlas_arm_gravload_minvarpar/1, atlas_arm_coriolis_vec_minvarpar/1, atlas_joint_impctrl_sqrt_damping_base/1, atlas_arm_inertia_minvarpar/1
  qD/1 -> momentum_based_friction_observer/5, atlas_arm_coriolis_vec_minvarpar/2, atlas_joint_impctrl_sqrt_damping_base/2
  q_d/1 -> atlas_joint_impctrl_sqrt_damping_base/3
  atlas_arm_coriolis_vec_minvarpar/1 -> momentum_based_friction_observer/4, atlas_joint_impctrl_sqrt_damping_base/6
  qD_d/1 -> atlas_joint_impctrl_sqrt_damping_base/4
  atlas_arm_gravload_minvarpar/1 -> momentum_based_friction_observer/3, atlas_joint_impctrl_sqrt_damping_base/7
  qDD_d/1 -> atlas_joint_impctrl_sqrt_damping_base/5
  g/1 -> atlas_arm_gravload_minvarpar/2
  momentum_based_friction_observer/1 -> atlas_joint_impctrl_sqrt_damping_base/9, tau_fr_obs/1
  tau_J/1 -> momentum_based_friction_observer/1
  tau_ext/1 -> momentum_based_friction_observer/2

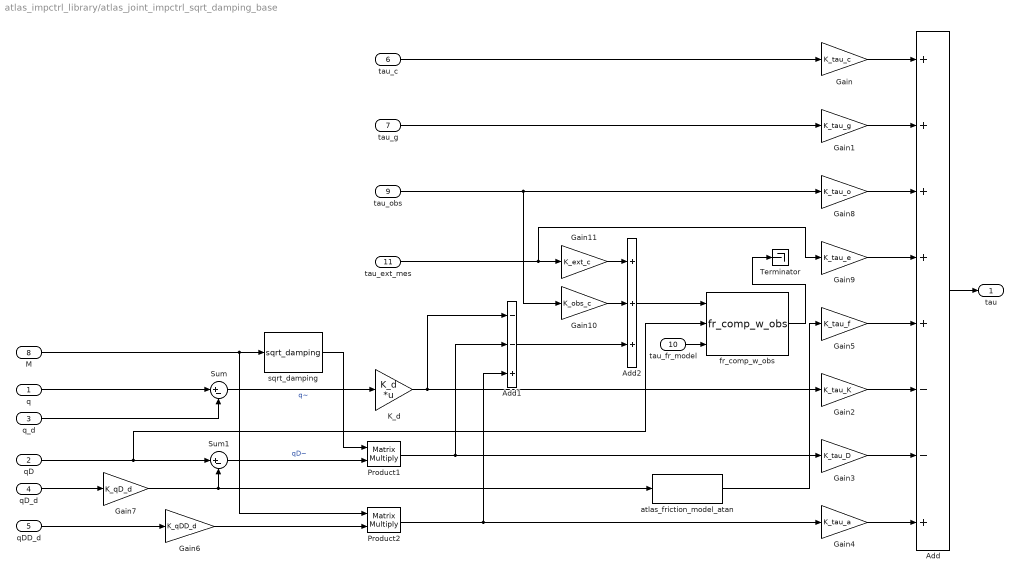
== system atlas_impctrl_library/atlas_joint_impctrl_sqrt_damping_base ==
  q : Inport
  qD : Inport  Port=2
  q_d : Inport  Port=3
  qD_d : Inport  Port=4
  qDD_d : Inport  Port=5
  tau_c : Inport  Port=6
  tau_g : Inport  Port=7
  M : Inport  Port=8
  tau_obs : Inport  Port=9
  tau_fr_model : Inport  Port=10
  tau_ext_mes : Inport  Port=11
  Add : Sum  Inputs=+++++--+
  Add1 : Sum  Inputs=--+
  Add2 : Sum  Inputs=+++
  Gain : Gain  Gain=K_tau_c
  Gain1 : Gain  Gain=K_tau_g
  Gain10 : Gain  Gain=K_obs_c
  Gain11 : Gain  Gain=K_ext_c
  Gain2 : Gain  Gain=K_tau_K
  Gain3 : Gain  Gain=K_tau_D
  Gain4 : Gain  Gain=K_tau_a
  Gain5 : Gain  Gain=K_tau_f
  Gain6 : Gain  Gain=K_qDD_d
  Gain7 : Gain  Gain=K_qD_d
  Gain8 : Gain  Gain=K_tau_o
  Gain9 : Gain  Gain=K_tau_e
  K_d : Gain  Gain=K_d  Multiplication=Matrix(K*u)
  Product1 : Product  Multiplication=Matrix(*)
  Product2 : Product  Multiplication=Matrix(*)
  Sum : Sum  Inputs=|+-
  Sum1 : Sum  Inputs=|+-
  Terminator : Terminator
  atlas_friction_model_atan : atlas_impctrl_library/atlas_friction_model_atan  tau_c=tau_c  B=B
  fr_comp_w_obs : atlas_impctrl_library/fr_comp_w_obs  tau_c=tau_c  B=B  qD_th=qD_th  tau_th=tau_th
  sqrt_damping : atlas_impctrl_library/sqrt_damping  K_d=K_d  D=D
  tau : Outport
  wires:
  Gain6/1 -> Product2/2
  Gain7/1 -> Sum1/2, atlas_friction_model_atan/1
  q_d/1 -> Sum/2
  M/1 -> Product2/1, sqrt_damping/1
  q/1 -> Sum/1
  qD/1 -> fr_comp_w_obs/2, Sum1/1
  qD_d/1 -> Gain7/1
  Sum1/1 -> Product1/2  "qD~"
  Sum/1 -> K_d/1  "q~"
  qDD_d/1 -> Gain6/1
  sqrt_damping/1 -> Product1/1
  Add/1 -> tau/1
  K_d/1 -> Gain2/1, Add1/1
  tau_g/1 -> Gain1/1
  tau_c/1 -> Gain/1
  Product1/1 -> Gain3/1, Add1/2
  Product2/1 -> Gain4/1, Add1/3
  Gain/1 -> Add/1
  Gain1/1 -> Add/2
  fr_comp_w_obs/1 -> Terminator/1
  tau_obs/1 -> Gain8/1, Gain10/1
  tau_fr_model/1 -> fr_comp_w_obs/3
  Gain5/1 -> Add/5
  Gain2/1 -> Add/6
  Gain3/1 -> Add/7
  Gain4/1 -> Add/8
  Gain8/1 -> Add/3
  tau_ext_mes/1 -> Gain9/1, Gain11/1
  Gain9/1 -> Add/4
  Add2/1 -> fr_comp_w_obs/1
  Add1/1 -> Add2/3
  Gain10/1 -> Add2/2
  Gain11/1 -> Add2/1
  atlas_friction_model_atan/1 -> Gain5/1

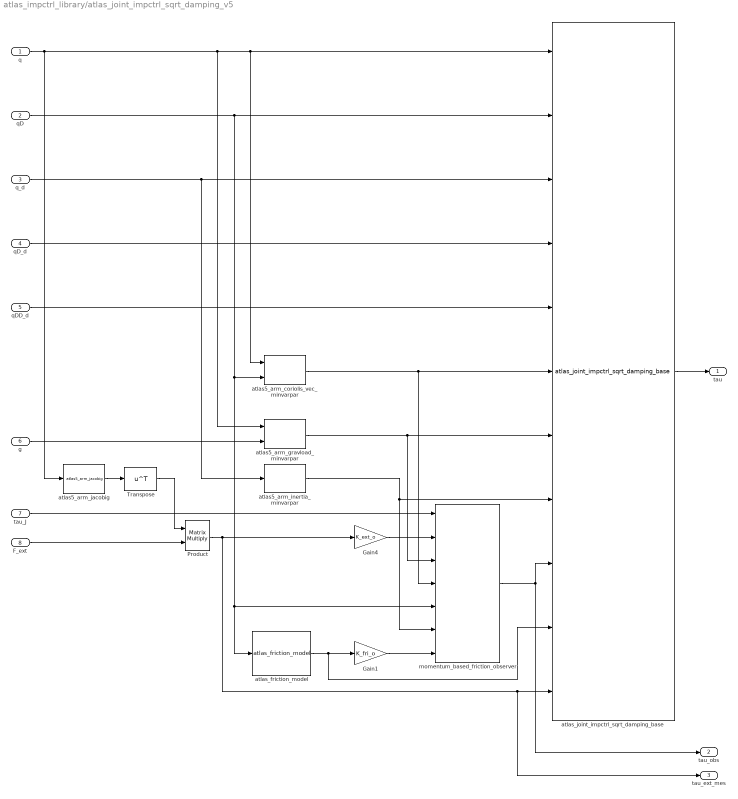
== system atlas_impctrl_library/atlas_joint_impctrl_sqrt_damping_v5 ==
  q : Inport  OutDataTypeStr=double  PortDimensions=7
  qD : Inport  Port=2  OutDataTypeStr=double  PortDimensions=7
  q_d : Inport  Port=3  OutDataTypeStr=double  PortDimensions=7
  qD_d : Inport  Port=4  OutDataTypeStr=double  PortDimensions=7
  qDD_d : Inport  Port=5  OutDataTypeStr=double  PortDimensions=7
  g : Inport  Port=6  OutDataTypeStr=double  PortDimensions=3
  tau_J : Inport  Port=7  OutDataTypeStr=double  PortDimensions=7
  F_ext : Inport  Port=8  OutDataTypeStr=double  PortDimensions=6
  Gain1 : Gain  Gain=K_fri_o
  Gain4 : Gain  Gain=K_ext_o
  Product : Product  Multiplication=Matrix(*)
  Transpose : Math  Operator=transpose  SaturateOnIntegerOverflow=on
  atlas5_arm_coriolis_vec_minvarpar : atlas_dynamic_library/atlas5_arm_coriolis_vec_minvarpar  atlas_arm_lr=atlas_arm_lr  MPV=MPV_arm_model
  atlas5_arm_gravload_minvarpar : atlas_dynamic_library/atlas5_arm_gravload_minvarpar  atlas_arm_lr=atlas_arm_lr  MPV=MPV_arm_model
  atlas5_arm_inertia_minvarpar : atlas_dynamic_library/atlas5_arm_inertia_minvarpar  atlas_arm_lr=atlas_arm_lr  MPV=MPV_arm_damp
  atlas5_arm_jacobig : atlas_dynamic_library/atlas5_arm_jacobig
  atlas_friction_model : atlas_impctrl_library/atlas_friction_model  tau_c=tau_c  B=B
  atlas_joint_impctrl_sqrt_damping_base : atlas_impctrl_library/atlas_joint_impctrl_sqrt_damping_base  K_d=K_d  D=D  K_tau_g=K_tau_g  K_tau_c=K_tau_c  K_tau_K=K_tau_K  K_tau_D=K_tau_D  K_tau_a=K_tau_a  K_tau_f=K_tau_f  K_tau_e=K_tau_e  K_tau_o=K_tau_o  K_qD_d=K_qD_d  K_qDD_d=K_qDD_d  K_ext_c=K_ext_c  K_obs_c=K_obs_c  tau_c=tau_c  B=B  qD_th=qD_th  tau_th=tau_th
  momentum_based_friction_observer : atlas_impctrl_library/momentum_based_friction_observer  K_O=K_O  T=T  T1=T1  tau_out_max=tau_obs_max
  tau : Outport  OutDataTypeStr=double  PortDimensions=7
  tau_obs : Outport  Port=2  OutDataTypeStr=double  PortDimensions=7
  tau_ext_mes : Outport  Port=3  OutDataTypeStr=double  PortDimensions=7
  wires:
  atlas_joint_impctrl_sqrt_damping_base/1 -> tau/1
  atlas5_arm_inertia_minvarpar/1 -> momentum_based_friction_observer/6, atlas_joint_impctrl_sqrt_damping_base/8
  q/1 -> atlas5_arm_jacobig/1, atlas5_arm_gravload_minvarpar/1, atlas5_arm_coriolis_vec_minvarpar/1, atlas_joint_impctrl_sqrt_damping_base/1
  qD/1 -> atlas_joint_impctrl_sqrt_damping_base/2, atlas5_arm_coriolis_vec_minvarpar/2, atlas_friction_model/1, momentum_based_friction_observer/5
  q_d/1 -> atlas5_arm_inertia_minvarpar/1, atlas_joint_impctrl_sqrt_damping_base/3
  atlas5_arm_coriolis_vec_minvarpar/1 -> momentum_based_friction_observer/4, atlas_joint_impctrl_sqrt_damping_base/6
  qD_d/1 -> atlas_joint_impctrl_sqrt_damping_base/4
  atlas5_arm_gravload_minvarpar/1 -> momentum_based_friction_observer/3, atlas_joint_impctrl_sqrt_damping_base/7
  qDD_d/1 -> atlas_joint_impctrl_sqrt_damping_base/5
  g/1 -> atlas5_arm_gravload_minvarpar/2
  momentum_based_friction_observer/1 -> tau_obs/1, atlas_joint_impctrl_sqrt_damping_base/9
  tau_J/1 -> momentum_based_friction_observer/1
  atlas5_arm_jacobig/1 -> Transpose/1
  Transpose/1 -> Product/1
  F_ext/1 -> Product/2
  Product/1 -> tau_ext_mes/1, atlas_joint_impctrl_sqrt_damping_base/11, Gain4/1
  atlas_friction_model/1 -> atlas_joint_impctrl_sqrt_damping_base/10, Gain1/1
  Gain4/1 -> momentum_based_friction_observer/2
  Gain1/1 -> momentum_based_friction_observer/7

== system atlas_impctrl_library/atlas_joint_impctrl_v5 ==
  q : Inport
  qD : Inport  Port=2
  q_d : Inport  Port=3
  qD_d : Inport  Port=4
  qDD_d : Inport  Port=5
  g : Inport  Port=6
  atlas_arm_coriolis_vec_minvarpar : atlas_dynamic_library/atlas_arm_coriolis_vec_minvarpar  atlas_arm_lr=atlas_arm_lr  atlas_version=atlas_version  MPV=MPV
  atlas_arm_gravload_minvarpar : atlas_dynamic_library/atlas_arm_gravload_minvarpar  atlas_arm_lr=atlas_arm_lr  atlas_version=atlas_version  MPV=MPV
  atlas_arm_inertia_minvarpar : atlas_dynamic_library/atlas_arm_inertia_minvarpar  atlas_arm_lr=atlas_arm_lr  atlas_version=atlas_version  MPV=MPV
  atlas_joint_impctrl_base : atlas_impctrl_library/atlas_joint_impctrl_base  K_d=K_d  D=D  tau_c=tau_c  B=B  tau_s=tau_s  qD_s=qD_s  delta_s=delta_s  qD_th=qD_th  tau_th=tau_th  K_tau_g=K_tau_g  K_tau_c=K_tau_c  K_tau_F=K_tau_F  K_tau_K=K_tau_K  K_tau_D=K_tau_D  K_tau_a=K_tau_a
  tau : Outport
  wires:
  atlas_joint_impctrl_base/1 -> tau/1
  atlas_arm_inertia_minvarpar/1 -> atlas_joint_impctrl_base/8
  q/1 -> atlas_arm_inertia_minvarpar/1, atlas_arm_gravload_minvarpar/1, atlas_joint_impctrl_base/1, atlas_arm_coriolis_vec_minvarpar/1
  qD/1 -> atlas_joint_impctrl_base/2, atlas_arm_coriolis_vec_minvarpar/2
  q_d/1 -> atlas_joint_impctrl_base/3
  atlas_arm_coriolis_vec_minvarpar/1 -> atlas_joint_impctrl_base/6
  qD_d/1 -> atlas_joint_impctrl_base/4
  atlas_arm_gravload_minvarpar/1 -> atlas_joint_impctrl_base/7
  qDD_d/1 -> atlas_joint_impctrl_base/5
  g/1 -> atlas_arm_gravload_minvarpar/2

== system atlas_impctrl_library/compensate_hand_mass_and_offset ==
  W_raw : Inport
  g_hand : Inport  Port=2
  compensate_hand_mass_and_offset : MATLAB Function  TreatAsAtomicUnit=on
  W_comp : Outport
  wires:
  W_raw/1 -> compensate_hand_mass_and_offset/1(W_raw)
  g_hand/1 -> compensate_hand_mass_and_offset/2(g_hand)
  compensate_hand_mass_and_offset/1(W_comp) -> W_comp/1

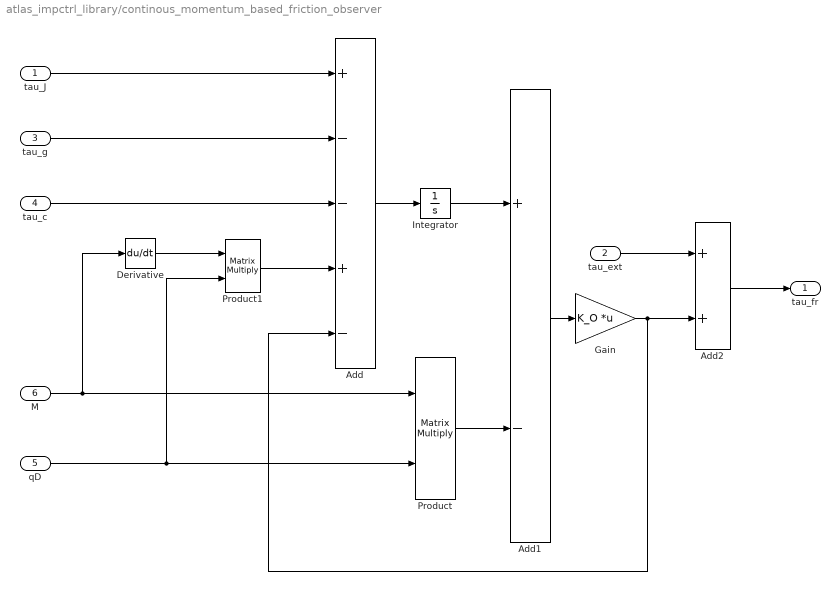
== system atlas_impctrl_library/continous_momentum_based_friction_observer ==
  tau_J : Inport
  tau_ext : Inport  Port=2
  tau_g : Inport  Port=3
  tau_c : Inport  Port=4
  qD : Inport  Port=5
  M : Inport  Port=6
  Add : Sum  Inputs=+--+-
  Add1 : Sum  Inputs=+-
  Add2 : Sum
  Derivative : Derivative
  Gain : Gain  Gain=K_O  Multiplication=Matrix(K*u)
  Integrator : Integrator
  Product : Product  Multiplication=Matrix(*)
  Product1 : Product  Multiplication=Matrix(*)
  tau_fr : Outport
  wires:
  Add/1 -> Integrator/1
  Integrator/1 -> Add1/1
  Product/1 -> Add1/2
  M/1 -> Derivative/1, Product/1
  qD/1 -> Product1/2, Product/2
  Derivative/1 -> Product1/1
  Add1/1 -> Gain/1
  Gain/1 -> Add/5, Add2/2
  Product1/1 -> Add/4
  tau_J/1 -> Add/1
  tau_g/1 -> Add/2
  tau_c/1 -> Add/3
  Add2/1 -> tau_fr/1
  tau_ext/1 -> Add2/1

== system atlas_impctrl_library/double_diag ==
  M : Inport
  MATLAB double_diag : MATLAB Function  TreatAsAtomicUnit=on
  D_d : Outport
  wires:
  M/1 -> MATLAB double_diag/1(M)
  MATLAB double_diag/1(D_d) -> D_d/1

== system atlas_impctrl_library/fr_comp_w_obs ==
  tau_imp : Inport
  qD : Inport  Port=2
  tau_fr_model : Inport  Port=3
  MATLAB fr_comp_w_obs : MATLAB Function  TreatAsAtomicUnit=on
  tau_F : Outport
  wires:
  qD/1 -> MATLAB fr_comp_w_obs/2(qD)
  MATLAB fr_comp_w_obs/1(tau_F) -> tau_F/1
  tau_imp/1 -> MATLAB fr_comp_w_obs/1(tau_imp)
  tau_fr_model/1 -> MATLAB fr_comp_w_obs/3(tau_fr_model)

== system atlas_impctrl_library/friction_compensation ==
  tau_imp : Inport
  qD : Inport  Port=2
  MATLAB sqrt_damping : MATLAB Function  TreatAsAtomicUnit=on
  tau_F : Outport
  wires:
  qD/1 -> MATLAB sqrt_damping/2(qD)
  MATLAB sqrt_damping/1(tau_F) -> tau_F/1
  tau_imp/1 -> MATLAB sqrt_damping/1(tau_imp)

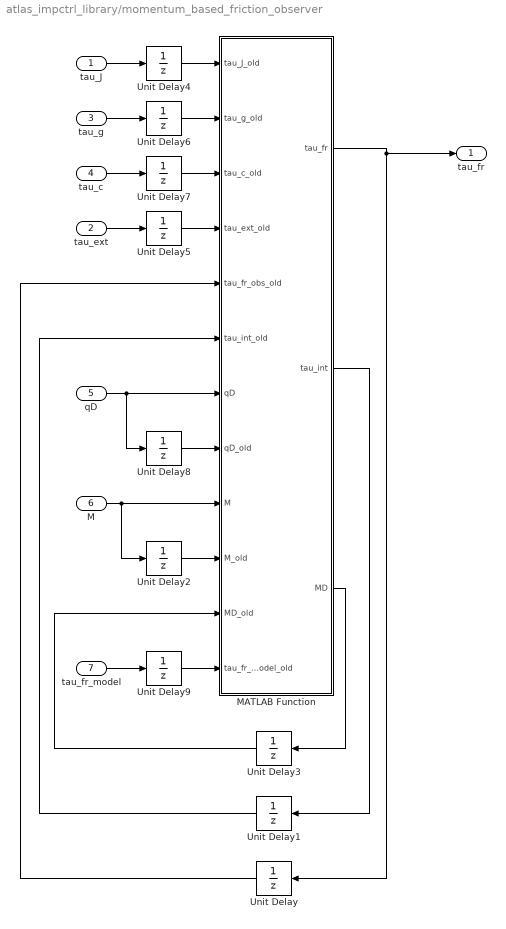
== system atlas_impctrl_library/momentum_based_friction_observer ==
  tau_J : Inport  OutDataTypeStr=double
  tau_ext : Inport  Port=2  OutDataTypeStr=double
  tau_g : Inport  Port=3  OutDataTypeStr=double
  tau_c : Inport  Port=4  OutDataTypeStr=double
  qD : Inport  Port=5  OutDataTypeStr=double
  M : Inport  Port=6  OutDataTypeStr=double
  tau_fr_model : Inport  Port=7  OutDataTypeStr=double
  MATLAB Function : MATLAB Function  TreatAsAtomicUnit=on
  Unit Delay{,1..9} (10 alike) : UnitDelay  SampleTime=-1
  tau_fr : Outport  OutDataTypeStr=double
  wires:
  Unit Delay/1 -> MATLAB Function/5(tau_fr_obs_old)
  tau_g/1 -> Unit Delay6/1
  tau_J/1 -> Unit Delay4/1
  M/1 -> Unit Delay2/1, MATLAB Function/9(M)
  qD/1 -> Unit Delay8/1, MATLAB Function/7(qD)
  tau_c/1 -> Unit Delay7/1
  MATLAB Function/2(tau_int) -> Unit Delay1/1
  Unit Delay1/1 -> MATLAB Function/6(tau_int_old)
  Unit Delay2/1 -> MATLAB Function/10(M_old)
  MATLAB Function/3(MD) -> Unit Delay3/1
  Unit Delay3/1 -> MATLAB Function/11(MD_old)
  Unit Delay4/1 -> MATLAB Function/1(tau_J_old)
  Unit Delay6/1 -> MATLAB Function/2(tau_g_old)
  Unit Delay7/1 -> MATLAB Function/3(tau_c_old)
  Unit Delay8/1 -> MATLAB Function/8(qD_old)
  MATLAB Function/1(tau_fr) -> Unit Delay/1, tau_fr/1
  tau_ext/1 -> Unit Delay5/1
  Unit Delay5/1 -> MATLAB Function/4(tau_ext_old)
  tau_fr_model/1 -> Unit Delay9/1
  Unit Delay9/1 -> MATLAB Function/12(tau_fr_model_old)

== system atlas_impctrl_library/sqrt_damping ==
  M : Inport
  MATLAB sqrt_damping : MATLAB Function  TreatAsAtomicUnit=on
  D_d : Outport
  wires:
  M/1 -> MATLAB sqrt_damping/1(M)
  MATLAB sqrt_damping/1(D_d) -> D_d/1

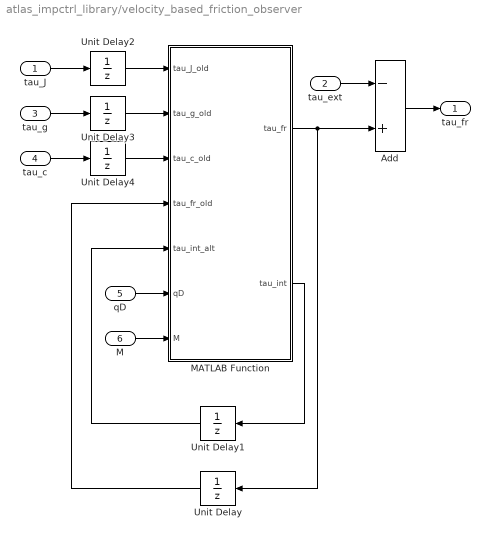
== system atlas_impctrl_library/velocity_based_friction_observer ==
  tau_J : Inport
  tau_ext : Inport  Port=2
  tau_g : Inport  Port=3
  tau_c : Inport  Port=4
  qD : Inport  Port=5
  M : Inport  Port=6
  Add : Sum  Inputs=-+
  MATLAB Function : MATLAB Function  TreatAsAtomicUnit=on
  Unit Delay{,1..4} (5 alike) : UnitDelay  SampleTime=-1
  tau_fr : Outport
  wires:
  MATLAB Function/1(tau_fr) -> Add/2, Unit Delay/1
  Unit Delay/1 -> MATLAB Function/4(tau_fr_old)
  tau_g/1 -> Unit Delay3/1
  tau_J/1 -> Unit Delay2/1
  M/1 -> MATLAB Function/7(M)
  qD/1 -> MATLAB Function/6(qD)
  tau_c/1 -> Unit Delay4/1
  tau_ext/1 -> Add/1
  MATLAB Function/2(tau_int) -> Unit Delay1/1
  Unit Delay1/1 -> MATLAB Function/5(tau_int_alt)
  Unit Delay2/1 -> MATLAB Function/1(tau_J_old)
  Unit Delay3/1 -> MATLAB Function/2(tau_g_old)
  Unit Delay4/1 -> MATLAB Function/3(tau_c_old)
  Add/1 -> tau_fr/1
